simulink model "sys3Tanks_v2"  (Simulink 7.7)
settings: Solver=ode4  StartTime=0.0  StopTime=300  FixedStep=0.01  RelTol=1e-3
values from neighbouring files (symbols this model uses):
  A = [-0.010464  0.010464  0; 0.010464  -0.021632  0.011168; 0  0.011168  -0.018598]    [datos.mat]    (also in parametros.mat)
  az1 = 0.511    [parametros.mat]
  az2 = 0.5279    [parametros.mat]
  az3 = 0.7313    [parametros.mat]
  dh1 = 1    [parametros.mat]
  dh2 = 0.2    [parametros.mat]
  dh3 = 0.05    [parametros.mat]
  g = 9.81    [parametros.mat]
  h1e = 0.6    [parametros.mat]
  h2e = 0.5    [parametros.mat]
  h3e = 0.4063002405    [parametros.mat]
  K = [0.0813857847622 5.38965016849 137.813424924]    [datos.mat]    (also in parametros.mat)
  kr = 146.982221925    [datos.mat]    (also in parametros.mat)
  L = [2315429.59762 449826.253813 122.95]    [datos.mat]    (also in parametros.mat)
  Q1e = 3.5787e-05    [parametros.mat]
  Q2e = 6.74495e-05    [parametros.mat]
  r = 0.4063002405    [parametros.mat]
  S = 0.0171    [parametros.mat]
  S1 = 5e-05    [parametros.mat]
  S2 = 5e-05    [parametros.mat]
  S3 = 5e-05    [parametros.mat]
libraries: simulink x2
settings Model: Creator=Victor  LastModifiedBy=Victor
settings DataIOCC: LimitDataPoints=off

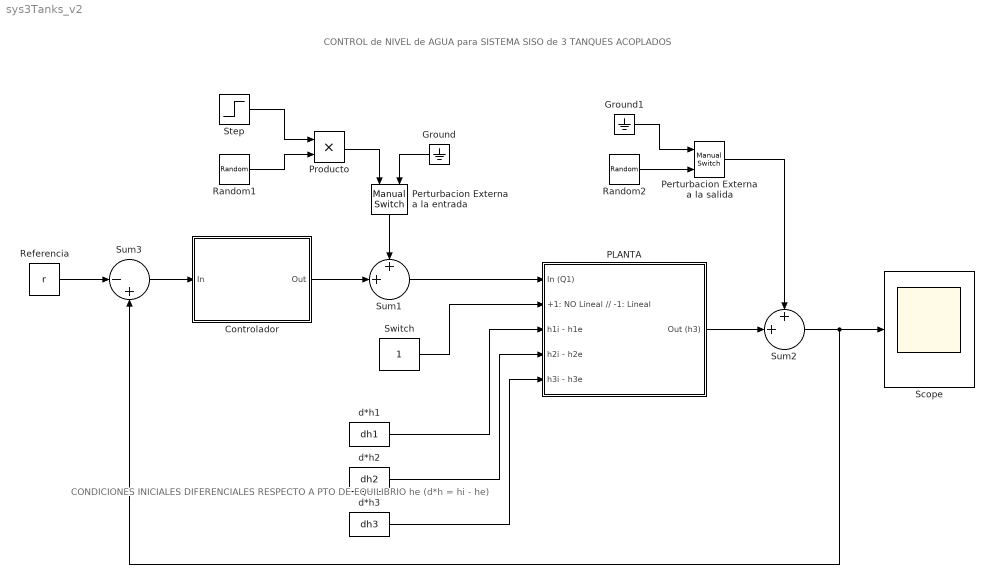
== system sys3Tanks_v2 ==
  note: CONTROL de NIVEL de AGUA para SISTEMA SISO de 3 TANQUES ACOPLADOS
  note: CONDICIONES INICIALES
      | DIFERENCIALES
      | RESPECTO A PTO
      | DE EQUILIBRIO he
      | (d*h = hi - he)
  Controlador : Subsystem  TreatAsAtomicUnit=on
  Ground : Ground
  Ground1 : Ground
  PLANTA : Subsystem  TreatAsAtomicUnit=on
  Perturbacion Externa a la entrada : simulink/Signal Routing/Manual Switch  SystemSampleTime=-1  sw=1  action=0  varsize=off
  Perturbacion Externa a la salida : simulink/Signal Routing/Manual Switch  SystemSampleTime=-1  sw=1  action=0  varsize=off
  Producto : Product  RndMeth=Zero
  Random1 : RandomNumber  Variance=5e-3
  Random2 : RandomNumber  Variance=5e-4
  Referencia : Constant  Value=r
  Scope : Scope
      settings: TimeRange=200  YMin=0  YMax=0.45
  Step : Step  Time=50  SampleTime=0
  Sum1 : Sum  Inputs=++|
  Sum2 : Sum  Inputs=++|
  Sum3 : Sum  Inputs=|-+
  Switch : Constant
  d*h1 : Constant  Value=dh1
  d*h2 : Constant  Value=dh2
  d*h3 : Constant  Value=dh3
  wires:
  Sum1/1 -> PLANTA/1(In (Q1))
  Sum2/1 -> Sum3/2, Scope/1
  PLANTA/1(Out (h3)) -> Sum2/2
  Referencia/1 -> Sum3/1
  Step/1 -> Producto/1
  Random1/1 -> Producto/2
  Perturbacion Externa a la salida/1 -> Sum2/1
  Perturbacion Externa a la entrada/1 -> Sum1/1
  Producto/1 -> Perturbacion Externa a la entrada/1
  Switch/1 -> PLANTA/2(+1: NO Lineal // -1: Lineal)
  d*h1/1 -> PLANTA/3(h1i - h1e)
  d*h2/1 -> PLANTA/4(h2i - h2e)
  d*h3/1 -> PLANTA/5(h3i - h3e)
  Controlador/1(Out) -> Sum1/2
  Ground/1 -> Perturbacion Externa a la entrada/2
  Random2/1 -> Perturbacion Externa a la salida/2
  Ground1/1 -> Perturbacion Externa a la salida/1
  Sum3/1 -> Controlador/1(In)

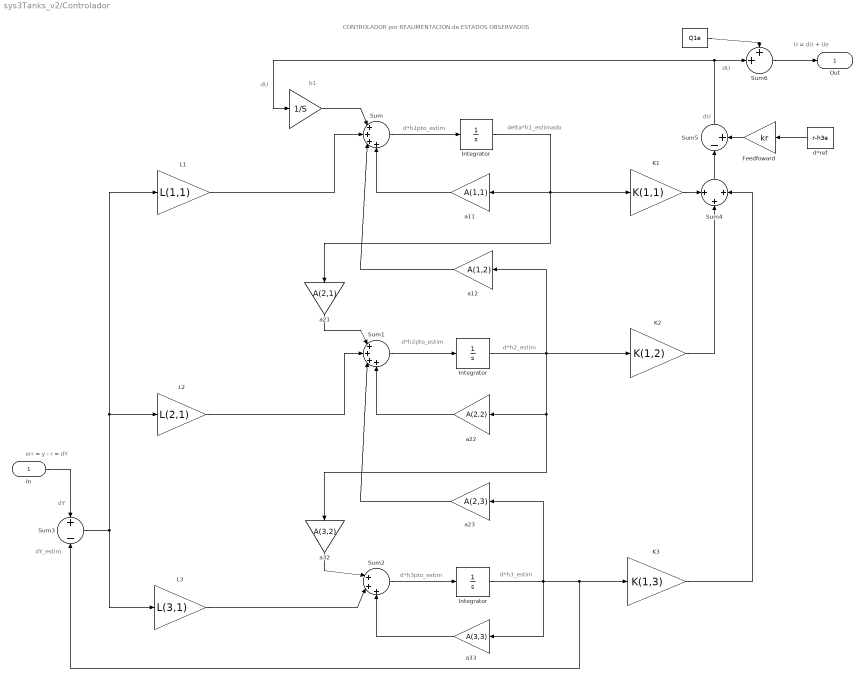
== system sys3Tanks_v2/Controlador ==
  note: dY_estim
  note: d*h1pto_estim
  note: delta*h1_estimado
  note: d*h2pto_estim
  note: d*h2_estim
  note: d*h3pto_estim
  note: d*h3_estim
  note: dU
  note: CONTROLADOR por REALIMENTACION de ESTADOS OBSERVADOS
  note: err = y - r = dY
  note: dY
  note: dU
  note: U = dU + Ue
  note: dU
  note: b1
  In : Inport
  " " : Constant  Value=Q1e
  "   " : Gain  Gain=1/S
  " Integrator " : Integrator
  Feedfoward : Gain  Gain=kr
  Integrator : Integrator
  "Integrator  " : Integrator
  K1 : Gain  Gain=K(1,1)
  K2 : Gain  Gain=K(1,2)
  K3 : Gain  Gain=K(1,3)
  L1 : Gain  Gain=L(1,1)
  L2 : Gain  Gain=L(2,1)
  L3 : Gain  Gain=L(3,1)
  Sum : Sum  Inputs=|++++
  Sum1 : Sum  Inputs=|++++
  Sum2 : Sum  Inputs=|+++
  Sum3 : Sum  Inputs=+|-
  Sum4 : Sum  Inputs=+|+|+
  Sum5 : Sum  Inputs=|-+
  Sum6 : Sum  Inputs=++|
  a11 : Gain  Gain=A(1,1)
  a12 : Gain  Gain=A(1,2)
  a21 : Gain  Gain=A(2,1)
  a22 : Gain  Gain=A(2,2)
  a23 : Gain  Gain=A(2,3)
  a32 : Gain  Gain=A(3,2)
  a33 : Gain  Gain=A(3,3)
  "d*ref  " : Constant  Value=r-h3e
  Out : Outport
  wires:
  Integrator/1 -> a11/1, K1/1, a21/1
  Sum/1 -> Integrator/1
  "   "/1 -> Sum/1
  "Integrator  "/1 -> a12/1, a22/1, a32/1, K2/1
  Sum1/1 -> "Integrator  "/1
  a21/1 -> Sum1/1
  " Integrator "/1 -> a33/1, a23/1, K3/1, Sum3/2
  Sum2/1 -> " Integrator "/1
  a32/1 -> Sum2/1
  Sum3/1 -> L2/1, L1/1, L3/1
  K1/1 -> Sum4/1
  K3/1 -> Sum4/3
  K2/1 -> Sum4/2
  Sum5/1 -> "   "/1, Sum6/2
  Feedfoward/1 -> Sum5/2
  "d*ref  "/1 -> Feedfoward/1
  Sum6/1 -> Out/1
  L3/1 -> Sum2/2
  a33/1 -> Sum2/3
  L2/1 -> Sum1/2
  a23/1 -> Sum1/3
  a22/1 -> Sum1/4
  L1/1 -> Sum/2
  a11/1 -> Sum/4
  a12/1 -> Sum/3
  " "/1 -> Sum6/1
  In/1 -> Sum3/1
  Sum4/1 -> Sum5/1

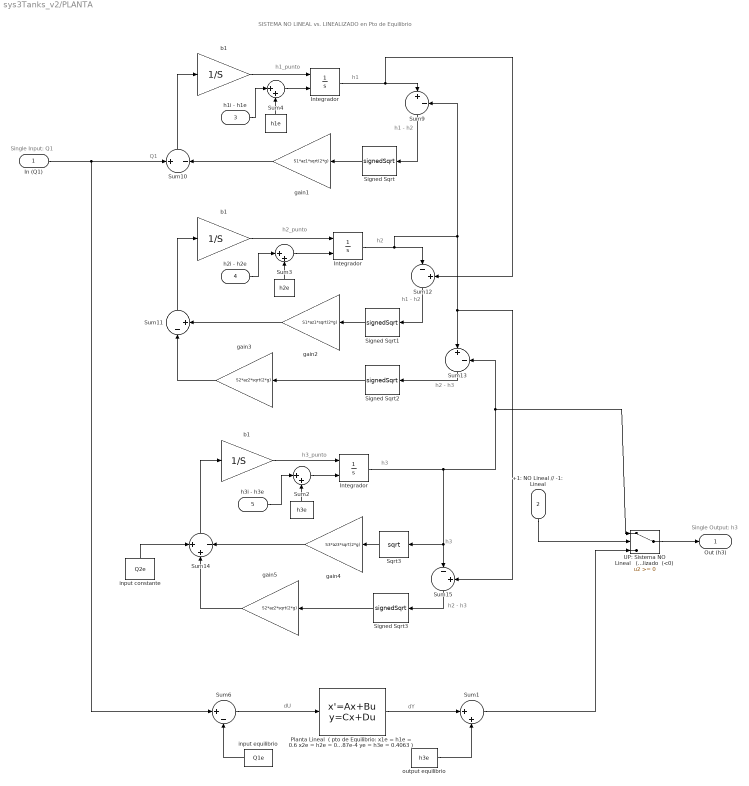
== system sys3Tanks_v2/PLANTA ==
  note: Q1
  note: h2 - h3
  note: h1 - h2
  note: h1 - h2
  note: h2 - h3
  note: h3
  note: h3
  note: h3_punto
  note: h2
  note: h2_punto
  note: h1_punto
  note: h1
  note: Single Input: Q1
  note: Single Output: h3
  note: SISTEMA NO LINEAL vs. LINEALIZADO en Pto de Equilibrio
  note: dU
  note: dY
  In (Q1) : Inport
  +1: NO Lineal // -1: Lineal : Inport  Port=2
  h1i - h1e : Inport  Port=3
  h2i - h2e : Inport  Port=4
  h3i - h3e : Inport  Port=5
  " " : Constant  Value=h1e
  "   " : Constant  Value=h2e
  "     " : Constant  Value=h3e
  " Integrador  " : Integrator  InitialConditionSource=external  InitialCondition=0.406
  " b1 " : Gain  Gain=1/S
  " input constante" : Constant  Value=Q2e
  Integrador : Integrator  InitialConditionSource=external  InitialCondition=0.5
  "Integrador " : Integrator  InitialConditionSource=external  InitialCondition=0.6
  Planta Lineal  ( pto de Equilibrio: x1e = h1e = 0.6 x2e = h2e = 0.5 x3e = h3e = 0.4063 ue = Q1e = 0.35787e-4 ye = h3e = 0.4063 ) : StateSpace  A=[-0.010464 0.010464 0; 0.010464 -0.021632 0.011168; 0 0.011168 -0.018598]  B=[58.4795; 0; 0]  C=[0 0 1]  D=0  X0=[0; 0; 0]
  Signed Sqrt{,1..3} (4 alike) : Sqrt  Operator=signedSqrt  SaturateOnIntegerOverflow=on
  Sqrt3 : Sqrt  OutputSignalType=real  SaturateOnIntegerOverflow=on
  Sum{1..4} (4 alike) : Sum  Inputs=|++
  Sum10 : Sum  Inputs=+|-
  Sum11 : Sum  Inputs=|-+
  Sum12 : Sum  Inputs=|-+
  Sum13 : Sum  Inputs=|+-
  Sum14 : Sum  Inputs=+|+|-
  Sum15 : Sum  Inputs=|-+
  Sum6 : Sum  Inputs=|+-
  Sum9 : Sum  Inputs=|+-
  UP: Sistema NO Lineal   (>=0) DOWN: Sistema Linealizado  (<0) : Switch
  b1 : Gain  Gain=1/S
  "b1   " : Gain  Gain=1/S
  gain1 : Gain  Gain=S1*az1*sqrt(2*g)
  gain2 : Gain  Gain=S1*az1*sqrt(2*g)
  gain3 : Gain  Gain=S2*az2*sqrt(2*g)
  gain4 : Gain  Gain=S3*az3*sqrt(2*g)
  gain5 : Gain  Gain=S2*az2*sqrt(2*g)
  input equilibrio : Constant  Value=Q1e
  output equilibrio : Constant  Value=h3e
  Out (h3) : Outport
  wires:
  "Integrador "/1 -> Sum12/2, Sum9/1
  b1/1 -> "Integrador "/1
  Sum10/1 -> b1/1
  Integrador/1 -> Sum12/1, Sum9/2, Sum13/1, Sum15/2
  "b1   "/1 -> Integrador/1
  Sum11/1 -> "b1   "/1
  " Integrador  "/1 -> Sum13/2, UP: Sistema NO Lineal   (>=0) DOWN: Sistema Linealizado  (<0)/1, Sum15/1, Sqrt3/1
  Sqrt3/1 -> gain4/1
  " b1 "/1 -> " Integrador  "/1
  Sum14/1 -> " b1 "/1
  gain4/1 -> Sum14/3
  Sum9/1 -> Signed Sqrt/1
  Signed Sqrt/1 -> gain1/1
  gain1/1 -> Sum10/2
  gain2/1 -> Sum11/2
  Signed Sqrt1/1 -> gain2/1
  Sum12/1 -> Signed Sqrt1/1
  Signed Sqrt2/1 -> gain3/1
  Sum13/1 -> Signed Sqrt2/1
  gain3/1 -> Sum11/1
  Sum15/1 -> Signed Sqrt3/1
  Signed Sqrt3/1 -> gain5/1
  gain5/1 -> Sum14/2
  " input constante"/1 -> Sum14/1
  input equilibrio/1 -> Sum6/2
  Sum6/1 -> Planta Lineal  ( pto de Equilibrio: x1e = h1e = 0.6 x2e = h2e = 0.5 x3e = h3e = 0.4063 ue = Q1e = 0.35787e-4 ye = h3e = 0.4063 )/1
  Planta Lineal  ( pto de Equilibrio: x1e = h1e = 0.6 x2e = h2e = 0.5 x3e = h3e = 0.4063 ue = Q1e = 0.35787e-4 ye = h3e = 0.4063 )/1 -> Sum1/1
  output equilibrio/1 -> Sum1/2
  In (Q1)/1 -> Sum10/1, Sum6/1
  Sum1/1 -> UP: Sistema NO Lineal   (>=0) DOWN: Sistema Linealizado  (<0)/3
  UP: Sistema NO Lineal   (>=0) DOWN: Sistema Linealizado  (<0)/1 -> Out (h3)/1
  +1: NO Lineal // -1: Lineal/1 -> UP: Sistema NO Lineal   (>=0) DOWN: Sistema Linealizado  (<0)/2
  Sum2/1 -> " Integrador  "/2
  "     "/1 -> Sum2/2
  h3i - h3e/1 -> Sum2/1
  "   "/1 -> Sum3/2
  Sum3/1 -> Integrador/2
  h2i - h2e/1 -> Sum3/1
  " "/1 -> Sum4/2
  h1i - h1e/1 -> Sum4/1
  Sum4/1 -> "Integrador "/2
